simulink model "test_on_intes_cross"  (R2019b)
settings: Solver=VariableStepAuto  StartTime=0.0  StopTime=inf  RelTol=1e-3
libraries: simulink x1
settings Model: Creator=lenovo  LastModifiedBy=lenovo

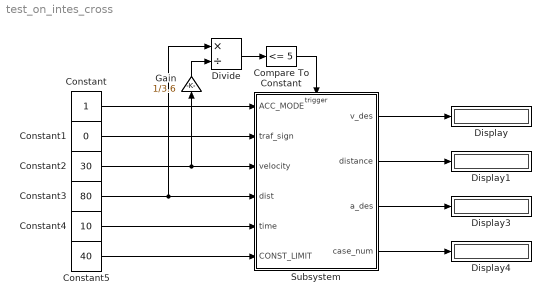
== system test_on_intes_cross ==
  Compare To Constant : simulink/Logic and Bit Operations/Compare To Constant  relop=<=  const=5  OutDataTypeStr=boolean
  Constant : Constant
  Constant1 : Constant  Value=0
  Constant2 : Constant  Value=30
  Constant3 : Constant  Value=80
  Constant4 : Constant  Value=10
  Constant5 : Constant  Value=40
  Display{,1,3..4} (4 alike) : Display
  Divide : Product  Inputs=*/
  Gain : Gain  Gain=1/3.6
  Subsystem : Subsystem
  wires:
  Constant/1 -> Subsystem/1(ACC_MODE)
  Constant1/1 -> Subsystem/2(traf_sign)
  Constant2/1 -> Subsystem/3(velocity), Gain/1
  Constant3/1 -> Divide/1, Subsystem/4(dist)
  Constant4/1 -> Subsystem/5(time)
  Constant5/1 -> Subsystem/6(CONST_LIMIT)
  Subsystem/1(v_des) -> Display/1
  Subsystem/2(distance) -> Display1/1
  Divide/1 -> Compare To Constant/1
  Subsystem/3(a_des) -> Display3/1
  Subsystem/4(case_num) -> Display4/1
  Compare To Constant/1 -> Subsystem/Trigger
  Gain/1 -> Divide/2

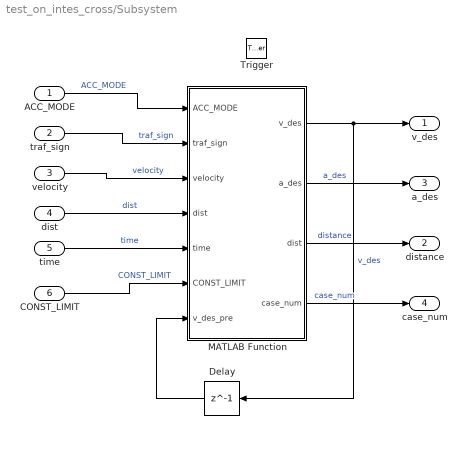
== system test_on_intes_cross/Subsystem ==
  ACC_MODE : Inport
  traf_sign : Inport  Port=2
  velocity : Inport  Port=3
  dist : Inport  Port=4
  time : Inport  Port=5
  CONST_LIMIT : Inport  Port=6
  Trigger : TriggerPort  VariantControl=Variant  PortDimensions=1
  Delay : Delay  DelayLength=1
  MATLAB Function : MATLAB Function  TreatAsAtomicUnit=on
  v_des : Outport
  distance : Outport  Port=2
  a_des : Outport  Port=3
  case_num : Outport  Port=4
  wires:
  velocity/1 -> MATLAB Function/3(velocity)  "velocity"
  CONST_LIMIT/1 -> MATLAB Function/6(CONST_LIMIT)  "CONST_LIMIT"
  traf_sign/1 -> MATLAB Function/2(traf_sign)  "traf_sign"
  MATLAB Function/3(dist) -> distance/1  "distance"
  MATLAB Function/1(v_des) -> Delay/1, v_des/1  "v_des"
  Delay/1 -> MATLAB Function/7(v_des_pre)
  dist/1 -> MATLAB Function/4("dist ")  "dist"
  ACC_MODE/1 -> MATLAB Function/1(ACC_MODE)  "ACC_MODE"
  time/1 -> MATLAB Function/5(time)  "time"
  MATLAB Function/2(a_des) -> a_des/1  "a_des"
  MATLAB Function/4(case_num) -> case_num/1  "case_num"

== matlab function test_on_intes_cross/Subsystem/MATLAB Function ==
  data: ACC_MODE input; v_des output; a_des output; traf_sign input; velocity input; dist input; time input; CONST_LIMIT input; dist output; v_des_pre input; case_num output

% clc
% clear all
% close all
% traf_sign = 0;
% velocity = 30;
% dist = 100;
% time = 12;
% CONST_LIMIT = 40;
% ACC_MODE = 0;

function [v_des,a_des,dist,case_num] = intesec_cross(ACC_MODE, traf_sign, velocity, dist, time,CONST_LIMIT,v_des_pre)  
%% this is a function that provide desired velocity, and distance to traffic light;
    % input: trafic_sign with green = 0; red = 1; yellow = 2;
    %        velocity in unit of kph;
    %        dist, and time is distance(m) to cross, and traffic time left
    %        CONST_LIMIT is velocity limit at cross, which is a reference CONSTANT velocity from
    %        ACC module.
    %        v_des_pre preseve previous v_des for next step use.
    
    % output: desired velocity for ACC module, in unit of kph;
    %         dist is distance(m) to front cross;
    
    green = 0;
    red = 1;
    yellow = 2;
    v = velocity / 3.6;
    distance = dist;
    CONST_LIMIT = CONST_LIMIT / 3.6;
    delta_t = 0.5;
    v_des = 0;
    a_des = 0;
    
    
    switch traf_sign
        case green
            if ACC_MODE == 0
                T = time;
                a = 2 * (dist - v * T) / (T^2 + 0.0001);
                v_temp = v + a * T;

                if (a >= 1) || ((a >= 0) && (a < 1) && (v_temp >= CONST_LIMIT))
                    v_des = 0;
                    a_des = 0;
                    case_num = 1;
                    
                elseif ((a < 0) && (v_temp >= 0) && (v_temp <= CONST_LIMIT))
                    v_des = CONST_LIMIT;
                    a_des = 0;
                    case_num = 2;
                else
                    v_des = v + a * T;
                    a_des = a;
                    case_num = 3;
                end
                
            else %(ACC_MODE == 1)
                T_ACC = dist / (v + 0.0001);
                if T_ACC < time - delta_t
                    v_des = v;
                    a_des = 0;
                    case_num = 4;
                    
                elseif T_ACC > time + delta_t
                    v_des = 0;
                    a_des = 0;
                    case_num = 5;
                    
                else
                    v_des = v_des_pre;
                    a_des = 0;
                    case_num = 6;
                end
            end
                          
        case red
            T = time + 1;
            a = 2 * (dist - v * T) / T^2;
            v_temp = v + a * T;
            
            
            if (a < -1)
                v_des = 0;
                a_des = 0;
                case_num = 7;
                
            elseif (a <=0 && a>= -1)
                v_des = v_temp;
                a_des = a;
                case_num = 8;
                
            elseif (a >= 0 && a <= 1 && v_temp < CONST_LIMIT)
                v_des = v_temp ; 
                a_des = a;
                case_num = 9;
                
            else
                v_des = CONST_LIMIT;
                a_des = 0;
                case_num = 10;
            end
       
    
                
        otherwise
            v_des = 0;
            a_des = 0;
            case_num = 11;
            
            
    end
    
    
    
    end
